simulink model "NonLinear_Nomoto1"  (R2015b)
settings: Solver=VariableStepAuto  StartTime=0.0  StopTime=tstop  FixedStep=0.01  RelTol=1e-3
values from neighbouring files (symbols this model uses):
  delta_c = dc_list(i)    [NonLinearAnalysis.m]    (also in Run_Delta_R_Sim.m = d_list(i); analyse_lin_dynamics.m = deg2rad(delta_list(i)); analyse_ulin_dynamics kopi.m = deg2rad(delta); analyse_ulin_dynamics.m = deg2rad(delta_list(i)))
  K = 0.0516730310612    [Heading_model.mat]    (also in Nomoto2_curvefitting.mat = 0.0627494534487; analyse_controller.m = place(A,B,P); analyse_lin_dynamics.m = x(2); analyse_ulin_dynamics kopi.m = x(2))
  T = x(1)    [analyse_lin_dynamics.m]    (also in analyse_ulin_dynamics kopi.m; analyse_ulin_dynamics.m; curvefitting.m = 1/x(1); run.m)
  tsamp = 10    [NonLinearAnalysis.m]    (also in analyse_lin_dynamics.m; analyse_steadystate.m; analyse_ulin_dynamics kopi.m; analyse_ulin_dynamics.m)
settings Model: Creator=Erik  LastModifiedBy=Erik
settings HardwareCC: ProdBitPerPointer=32  ProdLargestAtomicFloat=None  ProdIntDivRoundTo=Undefined  ProdEndianess=Unspecified  ProdWordSize=32  ProdHWDeviceType=32-bit Generic
settings GRTTargetCC: GeneratePreprocessorConditionals=Disable all

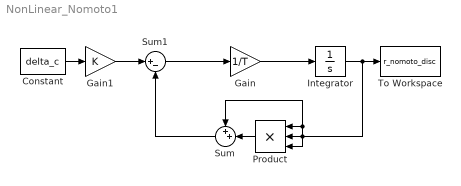
== system NonLinear_Nomoto1 ==
  Constant : Constant  Value=delta_c
  Gain : Gain  Gain=1/T
  Gain1 : Gain  Gain=K
  Integrator : Integrator
  Product : Product  Inputs=3
  Sum : Sum  Inputs=++|
  Sum1 : Sum  Inputs=|+-
  To Workspace : ToWorkspace  VariableName=r_nomoto_disc  SampleTime=tsamp
  wires:
  Gain/1 -> Integrator/1
  Constant/1 -> Gain1/1
  Integrator/1 -> To Workspace/1, Sum/1, Product/1, Product/3, Product/2
  Product/1 -> Sum/2
  Sum/1 -> Sum1/2
  Gain1/1 -> Sum1/1
  Sum1/1 -> Gain/1
